simulink model "bike_model_v1_20190513_oldmodel"  (R2016b)
settings: Solver=ode23s  StartTime=0.0  StopTime=sim_time  FixedStep=Ts_IMU  MaxStep=Ts  RelTol=1e-3
values from neighbouring files (symbols this model uses):
  A = [0      0            1 ... (first row only)    [bike_init_v1_20190523_oldmodel_NOfeedback_RealModelComparison.m]    (also in bike_init_v1_20190524_oldmodel_positionfeedback_Nobalancing.m; bike_init_v1_20190527_oldmodel_NObalancing.m; bike_init_v1_20190527_oldmodel_positionfeedback_and_indicator.m; bike_init_v1_20190528_oldmodel_positionfeedback_and_indicator.m)
  B = [0; 1; (a_real*v*sin(lambda_real))/(h_real*b_real)]    [bike_init_v1_20190523_oldmodel_NOfeedback_RealModelComparison.m]    (also in bike_init_v1_20190524_oldmodel_positionfeedback_Nobalancing.m; bike_init_v1_20190527_oldmodel_NObalancing.m; bike_init_v1_20190527_oldmodel_positionfeedback_and_indicator.m; bike_init_v1_20190528_oldmodel_positionfeedback_and_indicator.m)
  b_model = 1.095*(1+(-0.1+(0.2*rand)))    [bike_init_v1_20190523_oldmodel_NOfeedback_RealModelComparison.m]    (also in bike_init_v1_20190524_oldmodel_positionfeedback_Nobalancing.m = 1.095; bike_init_v1_20190527_oldmodel_NObalancing.m = 1.095; bike_init_v1_20190527_oldmodel_positionfeedback_and_indicator.m = 1.095; bike_init_v1_20190528_oldmodel_positionfeedback_and_indicator.m = 1.095)
  b_real = 1.095    [bike_init_v1_20190523_oldmodel_NOfeedback_RealModelComparison.m]    (also in bike_init_v1_20190524_oldmodel_positionfeedback_Nobalancing.m; bike_init_v1_20190527_oldmodel_NObalancing.m; bike_init_v1_20190527_oldmodel_positionfeedback_and_indicator.m; bike_init_v1_20190528_oldmodel_positionfeedback_and_indicator.m)
  complementary = 0.985    [bike_init_v1_20190523_oldmodel_NOfeedback_RealModelComparison.m]    (also in bike_init_v1_20190524_oldmodel_positionfeedback_Nobalancing.m; bike_init_v1_20190527_oldmodel_NObalancing.m; bike_init_v1_20190527_oldmodel_positionfeedback_and_indicator.m; bike_init_v1_20190528_oldmodel_positionfeedback_and_indicator.m)
  cumulative_dist_along_path = [0;cumsum(dist_from_vertex_to_vertex,1)]    [bike_init_v1_20190523_oldmodel_NOfeedback_RealModelComparison.m]    (also in bike_init_v1_20190524_oldmodel_positionfeedback_Nobalancing.m; bike_init_v1_20190527_oldmodel_NObalancing.m; bike_init_v1_20190527_oldmodel_positionfeedback_and_indicator.m; bike_init_v1_20190528_oldmodel_positionfeedback_and_indicator.m)
  damp = 0.4    [bike_init_v1_20190523_oldmodel_NOfeedback_RealModelComparison.m]    (also in bike_init_v1_20190524_oldmodel_positionfeedback_Nobalancing.m; bike_init_v1_20190527_oldmodel_NObalancing.m; bike_init_v1_20190527_oldmodel_positionfeedback_and_indicator.m; bike_init_v1_20190528_oldmodel_positionfeedback_and_indicator.m)
  Dead_Band = [0.055,-0.055,0.005]    [bike_init_v1_20190523_oldmodel_NOfeedback_RealModelComparison.m]    (also in bike_init_v1_20190524_oldmodel_positionfeedback_Nobalancing.m; bike_init_v1_20190527_oldmodel_NObalancing.m; bike_init_v1_20190527_oldmodel_positionfeedback_and_indicator.m; bike_init_v1_20190528_oldmodel_positionfeedback_and_indicator.m)
  delay = 0.045    [bike_init_v1_20190523_oldmodel_NOfeedback_RealModelComparison.m]    (also in bike_init_v1_20190524_oldmodel_positionfeedback_Nobalancing.m; bike_init_v1_20190527_oldmodel_NObalancing.m; bike_init_v1_20190527_oldmodel_positionfeedback_and_indicator.m; bike_init_v1_20190528_oldmodel_positionfeedback_and_indicator.m)
  delta_control = 1    [bike_init_v1_20190523_oldmodel_NOfeedback_RealModelComparison.m]    (also in bike_init_v1_20190524_oldmodel_positionfeedback_Nobalancing.m; bike_init_v1_20190527_oldmodel_NObalancing.m; bike_init_v1_20190527_oldmodel_positionfeedback_and_indicator.m; bike_init_v1_20190528_oldmodel_positionfeedback_and_indicator.m)
  direct_control = 1    [bike_init_v1_20190523_oldmodel_NOfeedback_RealModelComparison.m]    (also in bike_init_v1_20190524_oldmodel_positionfeedback_Nobalancing.m; bike_init_v1_20190527_oldmodel_NObalancing.m; bike_init_v1_20190527_oldmodel_positionfeedback_and_indicator.m; bike_init_v1_20190528_oldmodel_positionfeedback_and_indicator.m)
  filter_model = 1    [bike_init_v1_20190523_oldmodel_NOfeedback_RealModelComparison.m]    (also in bike_init_v1_20190524_oldmodel_positionfeedback_Nobalancing.m; bike_init_v1_20190527_oldmodel_NObalancing.m; bike_init_v1_20190527_oldmodel_positionfeedback_and_indicator.m; bike_init_v1_20190528_oldmodel_positionfeedback_and_indicator.m)
  forward_motor_dynamics = 0    [bike_init_v1_20190523_oldmodel_NOfeedback_RealModelComparison.m]    (also in bike_init_v1_20190524_oldmodel_positionfeedback_Nobalancing.m; bike_init_v1_20190527_oldmodel_NObalancing.m; bike_init_v1_20190527_oldmodel_positionfeedback_and_indicator.m; bike_init_v1_20190528_oldmodel_positionfeedback_and_indicator.m)
  fr_oscil = 1    [bike_init_v1_20190523_oldmodel_NOfeedback_RealModelComparison.m]    (also in bike_init_v1_20190524_oldmodel_positionfeedback_Nobalancing.m; bike_init_v1_20190527_oldmodel_NObalancing.m; bike_init_v1_20190527_oldmodel_positionfeedback_and_indicator.m; bike_init_v1_20190528_oldmodel_positionfeedback_and_indicator.m)
  g = 9.81    [bike_init_v1_20190523_oldmodel_NOfeedback_RealModelComparison.m]    (also in bike_init_v1_20190524_oldmodel_positionfeedback_Nobalancing.m; bike_init_v1_20190527_oldmodel_NObalancing.m; bike_init_v1_20190527_oldmodel_positionfeedback_and_indicator.m; bike_init_v1_20190528_oldmodel_positionfeedback_and_indicator.m)
  gain = 0.3    [bike_init_v1_20190523_oldmodel_NOfeedback_RealModelComparison.m]    (also in bike_init_v1_20190524_oldmodel_positionfeedback_Nobalancing.m; bike_init_v1_20190527_oldmodel_NObalancing.m; bike_init_v1_20190527_oldmodel_positionfeedback_and_indicator.m; bike_init_v1_20190528_oldmodel_positionfeedback_and_indicator.m)
  IMU_height_model = 0.45*(1+(-0.1+(0.2*rand)))    [bike_init_v1_20190523_oldmodel_NOfeedback_RealModelComparison.m]    (also in bike_init_v1_20190524_oldmodel_positionfeedback_Nobalancing.m = 0.45; bike_init_v1_20190527_oldmodel_NObalancing.m = 0.45; bike_init_v1_20190527_oldmodel_positionfeedback_and_indicator.m = 0.45; bike_init_v1_20190528_oldmodel_positionfeedback_and_indicator.m = 0.45)
  IMU_height_real = 0.45    [bike_init_v1_20190523_oldmodel_NOfeedback_RealModelComparison.m]    (also in bike_init_v1_20190524_oldmodel_positionfeedback_Nobalancing.m; bike_init_v1_20190527_oldmodel_NObalancing.m; bike_init_v1_20190527_oldmodel_positionfeedback_and_indicator.m; bike_init_v1_20190528_oldmodel_positionfeedback_and_indicator.m)
  initial_states = [deg2rad(0) deg2rad(0) deg2rad(0)]    [bike_init_v1_20190523_oldmodel_NOfeedback_RealModelComparison.m]    (also in bike_init_v1_20190524_oldmodel_positionfeedback_Nobalancing.m; bike_init_v1_20190527_oldmodel_NObalancing.m; bike_init_v1_20190527_oldmodel_positionfeedback_and_indicator.m; bike_init_v1_20190528_oldmodel_positionfeedback_and_indicator.m = [deg2rad(1) deg2rad(0) deg2rad(0)])
  initial_x = path_x(1)+x_ini_diff    [bike_init_v1_20190523_oldmodel_NOfeedback_RealModelComparison.m]    (also in bike_init_v1_20190524_oldmodel_positionfeedback_Nobalancing.m; bike_init_v1_20190527_oldmodel_NObalancing.m; bike_init_v1_20190527_oldmodel_positionfeedback_and_indicator.m; bike_init_v1_20190528_oldmodel_positionfeedback_and_indicator.m)
  initial_y = radius+y_ini_diff    (= 20)    [bike_init_v1_20190523_oldmodel_NOfeedback_RealModelComparison.m]    (also in bike_init_v1_20190524_oldmodel_positionfeedback_Nobalancing.m; bike_init_v1_20190527_oldmodel_NObalancing.m; bike_init_v1_20190527_oldmodel_positionfeedback_and_indicator.m; bike_init_v1_20190528_oldmodel_positionfeedback_and_indicator.m)
  input_velocity = 2    [bike_init_v1_20190523_oldmodel_NOfeedback_RealModelComparison.m]    (also in bike_init_v1_20190524_oldmodel_positionfeedback_Nobalancing.m = 2.5; bike_init_v1_20190527_oldmodel_NObalancing.m = 2.5; bike_init_v1_20190527_oldmodel_positionfeedback_and_indicator.m = 3; bike_init_v1_20190528_oldmodel_positionfeedback_and_indicator.m = 7)
  K_full_dis = zeros(length(velocity_lqr),3)    [bike_init_v1_20190523_oldmodel_NOfeedback_RealModelComparison.m]    (also in bike_init_v1_20190524_oldmodel_positionfeedback_Nobalancing.m; bike_init_v1_20190527_oldmodel_NObalancing.m; bike_init_v1_20190527_oldmodel_positionfeedback_and_indicator.m; bike_init_v1_20190528_oldmodel_positionfeedback_and_indicator.m)
  lambda_model = deg2rad(70)*(1+(-0.1+(0.2*rand)))    [bike_init_v1_20190523_oldmodel_NOfeedback_RealModelComparison.m]    (also in bike_init_v1_20190524_oldmodel_positionfeedback_Nobalancing.m = deg2rad(70); bike_init_v1_20190527_oldmodel_NObalancing.m = deg2rad(70); bike_init_v1_20190527_oldmodel_positionfeedback_and_indicator.m = deg2rad(70); bike_init_v1_20190528_oldmodel_positionfeedback_and_indicator.m = deg2rad(70))
  lambda_real = deg2rad(70)    [bike_init_v1_20190523_oldmodel_NOfeedback_RealModelComparison.m]    (also in bike_init_v1_20190524_oldmodel_positionfeedback_Nobalancing.m; bike_init_v1_20190527_oldmodel_NObalancing.m; bike_init_v1_20190527_oldmodel_positionfeedback_and_indicator.m; bike_init_v1_20190528_oldmodel_positionfeedback_and_indicator.m)
  lat_control = 1    [bike_init_v1_20190523_oldmodel_NOfeedback_RealModelComparison.m]    (also in bike_init_v1_20190524_oldmodel_positionfeedback_Nobalancing.m; bike_init_v1_20190527_oldmodel_NObalancing.m; bike_init_v1_20190527_oldmodel_positionfeedback_and_indicator.m; bike_init_v1_20190528_oldmodel_positionfeedback_and_indicator.m)
  look_ahead = 0    [bike_init_v1_20190523_oldmodel_NOfeedback_RealModelComparison.m]    (also in bike_init_v1_20190524_oldmodel_positionfeedback_Nobalancing.m; bike_init_v1_20190527_oldmodel_NObalancing.m; bike_init_v1_20190527_oldmodel_positionfeedback_and_indicator.m; bike_init_v1_20190528_oldmodel_positionfeedback_and_indicator.m)
  max_handlebar = 40*(pi/180)    (= 0.698131700798)    [bike_init_v1_20190523_oldmodel_NOfeedback_RealModelComparison.m]    (also in bike_init_v1_20190524_oldmodel_positionfeedback_Nobalancing.m; bike_init_v1_20190527_oldmodel_NObalancing.m; bike_init_v1_20190527_oldmodel_positionfeedback_and_indicator.m; bike_init_v1_20190528_oldmodel_positionfeedback_and_indicator.m)
  max_roll = pi/2    (= 1.57079632679)    [bike_init_v1_20190523_oldmodel_NOfeedback_RealModelComparison.m]    (also in bike_init_v1_20190524_oldmodel_positionfeedback_Nobalancing.m; bike_init_v1_20190527_oldmodel_NObalancing.m; bike_init_v1_20190527_oldmodel_positionfeedback_and_indicator.m; bike_init_v1_20190528_oldmodel_positionfeedback_and_indicator.m)
  max_steering_motor_acc = inf    [bike_init_v1_20190523_oldmodel_NOfeedback_RealModelComparison.m]    (also in bike_init_v1_20190524_oldmodel_positionfeedback_Nobalancing.m; bike_init_v1_20190527_oldmodel_NObalancing.m; bike_init_v1_20190527_oldmodel_positionfeedback_and_indicator.m; bike_init_v1_20190528_oldmodel_positionfeedback_and_indicator.m)
  max_steering_motor_speed = 7.5    [bike_init_v1_20190523_oldmodel_NOfeedback_RealModelComparison.m]    (also in bike_init_v1_20190524_oldmodel_positionfeedback_Nobalancing.m; bike_init_v1_20190527_oldmodel_NObalancing.m; bike_init_v1_20190527_oldmodel_positionfeedback_and_indicator.m; bike_init_v1_20190528_oldmodel_positionfeedback_and_indicator.m)
  min_handlebar = -max_handlebar    (= -0.698131700798)    [bike_init_v1_20190523_oldmodel_NOfeedback_RealModelComparison.m]    (also in bike_init_v1_20190524_oldmodel_positionfeedback_Nobalancing.m; bike_init_v1_20190527_oldmodel_NObalancing.m; bike_init_v1_20190527_oldmodel_positionfeedback_and_indicator.m; bike_init_v1_20190528_oldmodel_positionfeedback_and_indicator.m)
  min_roll = - max_roll    (= -1.57079632679)    [bike_init_v1_20190523_oldmodel_NOfeedback_RealModelComparison.m]    (also in bike_init_v1_20190524_oldmodel_positionfeedback_Nobalancing.m; bike_init_v1_20190527_oldmodel_NObalancing.m; bike_init_v1_20190527_oldmodel_positionfeedback_and_indicator.m; bike_init_v1_20190528_oldmodel_positionfeedback_and_indicator.m)
  min_steering_motor_acc = -inf    [bike_init_v1_20190523_oldmodel_NOfeedback_RealModelComparison.m]    (also in bike_init_v1_20190524_oldmodel_positionfeedback_Nobalancing.m; bike_init_v1_20190527_oldmodel_NObalancing.m; bike_init_v1_20190527_oldmodel_positionfeedback_and_indicator.m; bike_init_v1_20190528_oldmodel_positionfeedback_and_indicator.m)
  min_steering_motor_speed = -7.5    [bike_init_v1_20190523_oldmodel_NOfeedback_RealModelComparison.m]    (also in bike_init_v1_20190524_oldmodel_positionfeedback_Nobalancing.m; bike_init_v1_20190527_oldmodel_NObalancing.m; bike_init_v1_20190527_oldmodel_positionfeedback_and_indicator.m; bike_init_v1_20190528_oldmodel_positionfeedback_and_indicator.m)
  noise = 1    [bike_init_v1_20190523_oldmodel_NOfeedback_RealModelComparison.m]    (also in bike_init_v1_20190524_oldmodel_positionfeedback_Nobalancing.m; bike_init_v1_20190527_oldmodel_NObalancing.m; bike_init_v1_20190527_oldmodel_positionfeedback_and_indicator.m; bike_init_v1_20190528_oldmodel_positionfeedback_and_indicator.m)
  noise_encoder = 1e-7    (= 1e-07)    [bike_init_v1_20190523_oldmodel_NOfeedback_RealModelComparison.m]    (also in bike_init_v1_20190524_oldmodel_positionfeedback_Nobalancing.m; bike_init_v1_20190527_oldmodel_NObalancing.m; bike_init_v1_20190527_oldmodel_positionfeedback_and_indicator.m; bike_init_v1_20190528_oldmodel_positionfeedback_and_indicator.m)
  noise_hall = 0    [bike_init_v1_20190523_oldmodel_NOfeedback_RealModelComparison.m]    (also in bike_init_v1_20190524_oldmodel_positionfeedback_Nobalancing.m = 0.01; bike_init_v1_20190527_oldmodel_NObalancing.m; bike_init_v1_20190527_oldmodel_positionfeedback_and_indicator.m = 0.01; bike_init_v1_20190528_oldmodel_positionfeedback_and_indicator.m = 0.01)
  oscillations_roll = 0    [bike_init_v1_20190523_oldmodel_NOfeedback_RealModelComparison.m]    (also in bike_init_v1_20190524_oldmodel_positionfeedback_Nobalancing.m; bike_init_v1_20190527_oldmodel_NObalancing.m; bike_init_v1_20190527_oldmodel_positionfeedback_and_indicator.m; bike_init_v1_20190528_oldmodel_positionfeedback_and_indicator.m)
  oscillations_steer = 0    [bike_init_v1_20190523_oldmodel_NOfeedback_RealModelComparison.m]    (also in bike_init_v1_20190524_oldmodel_positionfeedback_Nobalancing.m; bike_init_v1_20190527_oldmodel_NObalancing.m; bike_init_v1_20190527_oldmodel_positionfeedback_and_indicator.m; bike_init_v1_20190528_oldmodel_positionfeedback_and_indicator.m)
  parameters_model = [g h_model b_model a_model lambda_model c_model]    [bike_init_v1_20190523_oldmodel_NOfeedback_RealModelComparison.m]    (also in bike_init_v1_20190524_oldmodel_positionfeedback_Nobalancing.m; bike_init_v1_20190527_oldmodel_NObalancing.m; bike_init_v1_20190527_oldmodel_positionfeedback_and_indicator.m; bike_init_v1_20190528_oldmodel_positionfeedback_and_indicator.m)
  parameters_real = [g h_real b_real a_real lambda_real c_real]    [bike_init_v1_20190523_oldmodel_NOfeedback_RealModelComparison.m]    (also in bike_init_v1_20190524_oldmodel_positionfeedback_Nobalancing.m; bike_init_v1_20190527_oldmodel_NObalancing.m; bike_init_v1_20190527_oldmodel_positionfeedback_and_indicator.m; bike_init_v1_20190528_oldmodel_positionfeedback_and_indicator.m)
  path_tracking = 1    [bike_init_v1_20190523_oldmodel_NOfeedback_RealModelComparison.m]    (also in bike_init_v1_20190524_oldmodel_positionfeedback_Nobalancing.m; bike_init_v1_20190527_oldmodel_NObalancing.m; bike_init_v1_20190527_oldmodel_positionfeedback_and_indicator.m; bike_init_v1_20190528_oldmodel_positionfeedback_and_indicator.m = 0)
  path_x = [path_x1 path_x2 path_x3]    [bike_init_v1_20190523_oldmodel_NOfeedback_RealModelComparison.m]    (also in bike_init_v1_20190524_oldmodel_positionfeedback_Nobalancing.m; bike_init_v1_20190527_oldmodel_NObalancing.m; bike_init_v1_20190527_oldmodel_positionfeedback_and_indicator.m; bike_init_v1_20190528_oldmodel_positionfeedback_and_indicator.m)
  path_y = [path_y1 path_y2 path_y3]    [bike_init_v1_20190523_oldmodel_NOfeedback_RealModelComparison.m]    (also in bike_init_v1_20190524_oldmodel_positionfeedback_Nobalancing.m; bike_init_v1_20190527_oldmodel_NObalancing.m; bike_init_v1_20190527_oldmodel_positionfeedback_and_indicator.m; bike_init_v1_20190528_oldmodel_positionfeedback_and_indicator.m)
  plant_model = 1    [bike_init_v1_20190523_oldmodel_NOfeedback_RealModelComparison.m]    (also in bike_init_v1_20190524_oldmodel_positionfeedback_Nobalancing.m; bike_init_v1_20190527_oldmodel_NObalancing.m; bike_init_v1_20190527_oldmodel_positionfeedback_and_indicator.m; bike_init_v1_20190528_oldmodel_positionfeedback_and_indicator.m)
  roll_rate_coef = 0.9    [bike_init_v1_20190523_oldmodel_NOfeedback_RealModelComparison.m]    (also in bike_init_v1_20190524_oldmodel_positionfeedback_Nobalancing.m; bike_init_v1_20190527_oldmodel_NObalancing.m; bike_init_v1_20190527_oldmodel_positionfeedback_and_indicator.m; bike_init_v1_20190528_oldmodel_positionfeedback_and_indicator.m)
  sensordist = dout*pi/nrsensor    (= 0.439822971503)    [bike_init_v1_20190524_oldmodel_positionfeedback_Nobalancing.m]    (also in bike_init_v1_20190527_oldmodel_NObalancing.m; bike_init_v1_20190527_oldmodel_positionfeedback_and_indicator.m; bike_init_v1_20190528_oldmodel_positionfeedback_and_indicator.m; bike_init_v1_20190531_oldmodel_positionfeedback_and_indicator.m)
  steering_motor_limitations = 1    [bike_init_v1_20190523_oldmodel_NOfeedback_RealModelComparison.m]    (also in bike_init_v1_20190524_oldmodel_positionfeedback_Nobalancing.m; bike_init_v1_20190527_oldmodel_NObalancing.m; bike_init_v1_20190527_oldmodel_positionfeedback_and_indicator.m; bike_init_v1_20190528_oldmodel_positionfeedback_and_indicator.m)
  sys_con = ss(A,B,C,D)    [bike_init_v1_20190523_oldmodel_NOfeedback_RealModelComparison.m]    (also in bike_init_v1_20190524_oldmodel_positionfeedback_Nobalancing.m; bike_init_v1_20190527_oldmodel_NObalancing.m; bike_init_v1_20190527_oldmodel_positionfeedback_and_indicator.m; bike_init_v1_20190528_oldmodel_positionfeedback_and_indicator.m)
  sys_dis = c2d(sys_con,Ts)    [bike_init_v1_20190523_oldmodel_NOfeedback_RealModelComparison.m]    (also in bike_init_v1_20190524_oldmodel_positionfeedback_Nobalancing.m; bike_init_v1_20190527_oldmodel_NObalancing.m; bike_init_v1_20190527_oldmodel_positionfeedback_and_indicator.m; bike_init_v1_20190528_oldmodel_positionfeedback_and_indicator.m)
  ToleranceVelocityEst = 0.5    [bike_init_v1_20190524_oldmodel_positionfeedback_Nobalancing.m]    (also in bike_init_v1_20190527_oldmodel_NObalancing.m; bike_init_v1_20190527_oldmodel_positionfeedback_and_indicator.m; bike_init_v1_20190528_oldmodel_positionfeedback_and_indicator.m; bike_init_v1_20190531_oldmodel_positionfeedback_and_indicator.m)
  Ts = 0.04    [bike_init_v1_20190523_oldmodel_NOfeedback_RealModelComparison.m]    (also in bike_init_v1_20190524_oldmodel_positionfeedback_Nobalancing.m; bike_init_v1_20190527_oldmodel_NObalancing.m; bike_init_v1_20190527_oldmodel_positionfeedback_and_indicator.m; bike_init_v1_20190528_oldmodel_positionfeedback_and_indicator.m)
  Ts_IMU = 0.04    [bike_init_v1_20190523_oldmodel_NOfeedback_RealModelComparison.m]    (also in bike_init_v1_20190524_oldmodel_positionfeedback_Nobalancing.m; bike_init_v1_20190527_oldmodel_NObalancing.m; bike_init_v1_20190527_oldmodel_positionfeedback_and_indicator.m; bike_init_v1_20190528_oldmodel_positionfeedback_and_indicator.m)
  velocity_lqr = [velocity_lqr-0.1 velocity_lqr velocity_lqr+0.1]    [bike_init_v1_20190523_oldmodel_NOfeedback_RealModelComparison.m]    (also in bike_init_v1_20190524_oldmodel_positionfeedback_Nobalancing.m; bike_init_v1_20190527_oldmodel_NObalancing.m; bike_init_v1_20190527_oldmodel_positionfeedback_and_indicator.m; bike_init_v1_20190528_oldmodel_positionfeedback_and_indicator.m)
  velocity_wave_amp = 0.5    [bike_init_v1_20190523_oldmodel_NOfeedback_RealModelComparison.m]    (also in bike_init_v1_20190524_oldmodel_positionfeedback_Nobalancing.m; bike_init_v1_20190527_oldmodel_NObalancing.m; bike_init_v1_20190527_oldmodel_positionfeedback_and_indicator.m; bike_init_v1_20190528_oldmodel_positionfeedback_and_indicator.m)
  velocity_wave_freq = 0.3*2*pi    (= 1.88495559215)    [bike_init_v1_20190523_oldmodel_NOfeedback_RealModelComparison.m]    (also in bike_init_v1_20190524_oldmodel_positionfeedback_Nobalancing.m; bike_init_v1_20190527_oldmodel_NObalancing.m; bike_init_v1_20190527_oldmodel_positionfeedback_and_indicator.m; bike_init_v1_20190528_oldmodel_positionfeedback_and_indicator.m)
undefined symbols (not defined in the file or in its folder): curvature
libraries: simulink x13, dspsigops x2, simulink_extras x1
(part 1 of 3)
settings Model: Creator=Boaz Ash  LastModifiedBy=maximefeingesicht
settings DebuggingCC: UnconnectedInputMsg=none  UnconnectedOutputMsg=none  UnconnectedLineMsg=none

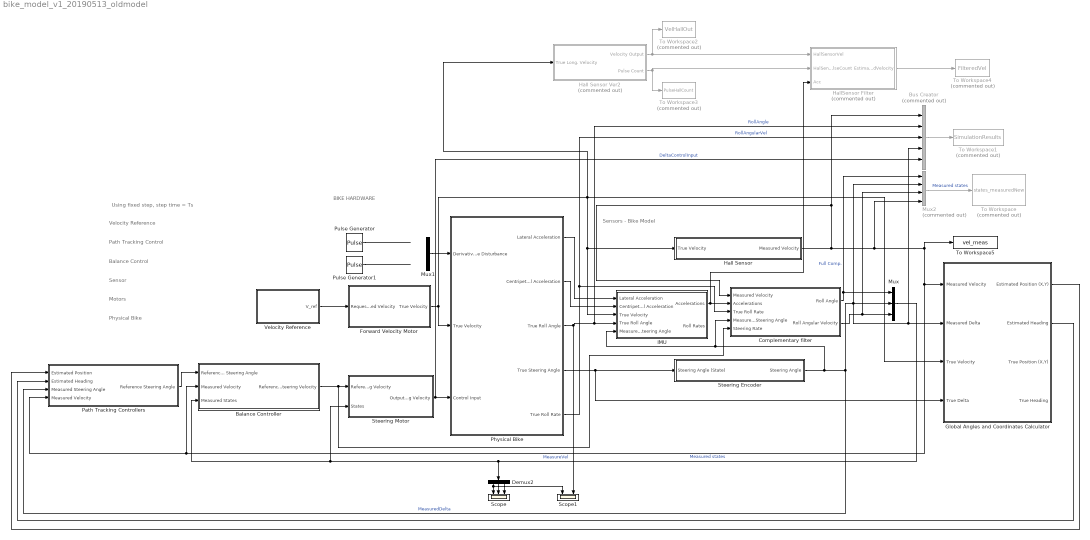
== system bike_model_v1_20190513_oldmodel ==
  note: Using fixed step, step time = Ts
  note: BIKE HARDWARE
  note: Velocity Reference
  note: Sensor
  note: Sensors - Bike Model
  note: Balance Control
  note: Motors
  note: Physical Bike
  note: Path Tracking Control
  Balance Controller : Subsystem  TreatAsAtomicUnit=on  SystemSampleTime=Ts
  Bus Creator : BusCreator  Commented=on  Inputs=5
  Complementary filter : Subsystem  SystemSampleTime=Ts_IMU
  Demux2 : Demux  Outputs=3
  Forward Velocity Motor : Subsystem
  Global Angles and Coordinates Calculator : Subsystem  SystemSampleTime=Ts
  Hall Sensor : Subsystem  TreatAsAtomicUnit=on  SystemSampleTime=Ts
  Hall Sensor Ver2 : Subsystem  Commented=on
  HallSensor Filter : Subsystem  Commented=on
  IMU : Subsystem  TreatAsAtomicUnit=on
  Mux : Mux  Inputs=3
  Mux1 : Mux  Inputs=3
  Mux2 : Mux  Commented=on
  Path Tracking Controllers : Subsystem
  Physical Bike : Subsystem
  Pulse Generator : DiscretePulseGenerator  PulseType=Time based  Amplitude=pi/36  Period=100  PhaseDelay=1
  Pulse Generator1 : DiscretePulseGenerator  PulseType=Time based  Amplitude=-deg2rad(30)  Period=10  PulseWidth=10  PhaseDelay=1
  Scope : Scope  NumInputPorts=3
  Scope1 : Scope  NumInputPorts=2
  Steering Encoder : Subsystem  TreatAsAtomicUnit=on  SystemSampleTime=Ts
  Steering Motor : Subsystem
  To Workspace : ToWorkspace  Commented=on  VariableName=states_measuredNew  SaveFormat=Timeseries  SampleTime=-1
  To Workspace1 : ToWorkspace  Commented=on  VariableName=SimulationResults  SaveFormat=Timeseries  SampleTime=-1
      settings: Decimation=2  Save2DSignal=2-D array (concatenate along first dimension)
  To Workspace2 : ToWorkspace  Commented=on  VariableName=VelHallOut  SaveFormat=Timeseries  SampleTime=Ts
  To Workspace3 : ToWorkspace  Commented=on  VariableName=PulseHallCount  SaveFormat=Timeseries  SampleTime=Ts
  To Workspace4 : ToWorkspace  Commented=on  VariableName=FilteredVel  SaveFormat=Timeseries  SampleTime=-1
  To Workspace5 : ToWorkspace  VariableName=vel_meas  SaveFormat=Timeseries  SampleTime=-1
  Velocity Reference : Subsystem
  wires:
  Complementary filter/1(Roll Angle) -> Mux2/1, Mux/1  "Full Comp."
  Complementary filter/2(Roll Angular Velocity) -> Mux2/3, Mux/3
  Mux1/1 -> Physical Bike/1(Derivative Disturbance)
  Velocity Reference/1(V_ref) -> Forward Velocity Motor/1(Requested Velocity)
  Demux2/2 -> Scope/2
  Demux2/3 -> Scope/3
  Forward Velocity Motor/1(True Velocity) -> Hall Sensor/1(True Velocity), IMU/3(True Velocity), Hall Sensor Ver2/1(True Long. Velocity), Global Angles and Coordinates Calculator/3(True Velocity), Physical Bike/2(True Velocity)
  Pulse Generator/1 -> ?
  Physical Bike/4(True Steering Angle) -> Global Angles and Coordinates Calculator/4(True Delta), Steering Encoder/1(Steering Angle (State))
  Pulse Generator1/1 -> ?
  Global Angles and Coordinates Calculator/1(Estimated Position (X,Y)) -> Path Tracking Controllers/1(Estimated Position)
  Global Angles and Coordinates Calculator/2(Estimated Heading) -> Path Tracking Controllers/2(Estimated Heading)
  Path Tracking Controllers/1(Reference Steering Angle) -> Balance Controller/1(Reference Steering Angle)
  Balance Controller/1(Reference Steering Velocity) -> Complementary filter/5(Steering Rate), Steering Motor/1(Reference Steering Velocity)
  Demux2/1 -> Scope1/1, Scope/1
  Physical Bike/1(Lateral Acceleration) -> IMU/1(Lateral Acceleration)
  Physical Bike/2(Centripetal Acceleration) -> IMU/2(Centripetal Acceleration)
  Mux2/1 -> To Workspace/1  "Measured states"
  Mux/1 -> Demux2/1, Steering Motor/2(States), Balance Controller/3(Measured States)  "Measured states"
  HallSensor Filter/1(EstimatedVelocity) -> To Workspace4/1
  Bus Creator/1 -> To Workspace1/1
  Hall Sensor/1(Measured Velocity) -> Bus Creator/1, Complementary filter/1(Measured Velocity), To Workspace5/1, Path Tracking Controllers/4(Measured Velocity), Balance Controller/2(Measured Velocity), Global Angles and Coordinates Calculator/1(Measured Velocity), Mux2/4  "MeasureVel"
  Physical Bike/5(True Roll Rate) -> Bus Creator/3, Complementary filter/3(True Roll Rate)  "RollAngularVel"
  Hall Sensor Ver2/1(Velocity Output) -> To Workspace2/1, HallSensor Filter/1(HallSensorVel)
  Physical Bike/3(True Roll Angle) -> Bus Creator/2, IMU/4(True Roll Angle), Scope1/2  "RollAngle"
  Steering Motor/1(Output Steering Velocity) -> Bus Creator/5, Physical Bike/3(Control Input)  "DeltaControlInput"
  Hall Sensor Ver2/2(" Pulse Count") -> HallSensor Filter/2(HalSensorPulseCount), To Workspace3/1
  Steering Encoder/1(Steering Angle) -> IMU/5(Measured Steering Angle), Complementary filter/4(Measured Steering Angle), Global Angles and Coordinates Calculator/2(Measured Delta), Bus Creator/4, Mux2/2, Mux/2, Path Tracking Controllers/3(Measured Steering Angle)  "MeasuredDelta"
  IMU/1(Accelerations) -> HallSensor Filter/3(Acc), Complementary filter/2(Accelerations)

== system bike_model_v1_20190513_oldmodel/Balance Controller ==
  Reference Steering Angle : Inport
  Measured Velocity : Inport  Port=2
  Measured States : Inport  Port=3
  LQR Controller : Subsystem  TreatAsAtomicUnit=on  SystemSampleTime=Ts
  Reference States : Subsystem  SystemSampleTime=Ts
  Sum : Sum  Inputs=|+-
  To Workspace : ToWorkspace  VariableName=states_measured  SaveFormat=Timeseries  SampleTime=-1
  Reference Steering Velocity : Outport
  wires:
  Reference States/1(Reference States) -> Sum/1
  Sum/1 -> LQR Controller/2(State Error)
  LQR Controller/1(Calculated Input) -> Reference Steering Velocity/1
  Reference Steering Angle/1 -> Reference States/2(Delta Ref)
  Measured Velocity/1 -> Reference States/1(Velocity), LQR Controller/1(Velocity)
  Measured States/1 -> To Workspace/1, Sum/2

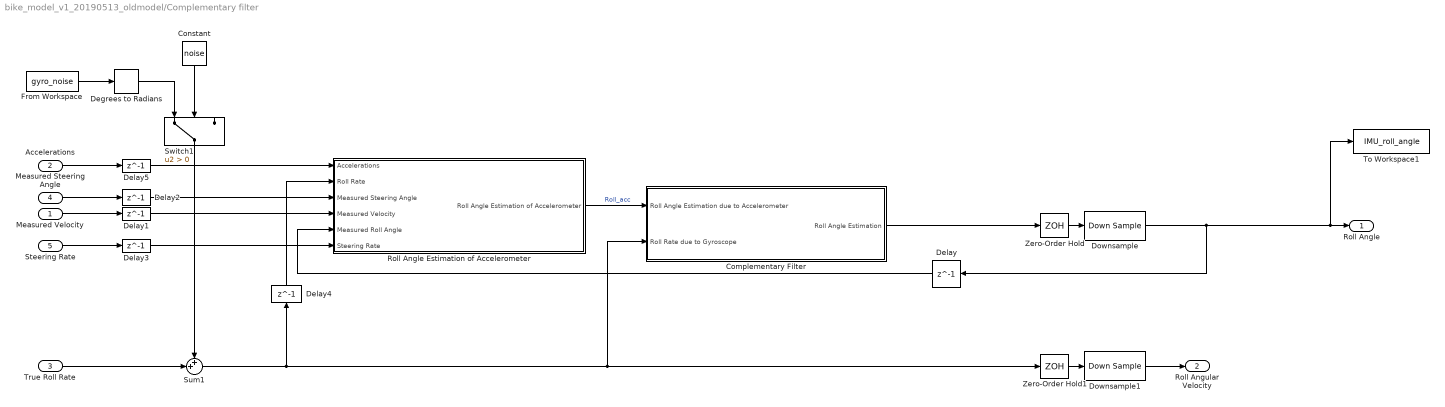
== system bike_model_v1_20190513_oldmodel/Complementary filter ==
  Measured Velocity : Inport
  Accelerations : Inport  Port=2
  True Roll Rate : Inport  Port=3
  Measured Steering Angle : Inport  Port=4
  Steering Rate : Inport  Port=5
  Complementary Filter : Subsystem  TreatAsAtomicUnit=on  SystemSampleTime=Ts_IMU
  Constant : Constant  Value=noise
  Degrees to Radians : simulink_extras/Transformations/Degrees to Radians
  Delay{,1..2,4..5} (5 alike) : Delay  DelayLength=1
  Delay3 : Delay  DelayLength=1  SampleTime=Ts_IMU
  Downsample : DownSample  N=Ts/Ts_IMU  RateOptions=Allow multirate processing
  Downsample1 : DownSample  N=Ts/Ts_IMU  RateOptions=Allow multirate processing
  From Workspace : FromWorkspace  VariableName=gyro_noise  SampleTime=0
  Roll Angle Estimation of Accelerometer : Subsystem
  Sum1 : Sum  Inputs=++|
  Switch1 : Switch  Criteria=u2 > Threshold
  To Workspace1 : ToWorkspace  VariableName=IMU_roll_angle  SaveFormat=Structure  SampleTime=-1
  Zero-Order Hold : ZeroOrderHold  SampleTime=Ts_IMU
  Zero-Order Hold1 : ZeroOrderHold  SampleTime=Ts_IMU
  Roll Angle : Outport
  Roll Angular Velocity : Outport  Port=2
  wires:
  Constant/1 -> Switch1/2
  True Roll Rate/1 -> Sum1/2
  Roll Angle Estimation of Accelerometer/1(Roll Angle Estimation of Accelerometer) -> Complementary Filter/1(Roll Angle Estimation due to Accelerometer)  "Roll_acc"
  Switch1/1 -> Sum1/1
  Sum1/1 -> Zero-Order Hold1/1, Complementary Filter/2(Roll Rate due to Gyroscope), Delay4/1
  Zero-Order Hold/1 -> Downsample/1
  Zero-Order Hold1/1 -> Downsample1/1
  Accelerations/1 -> Delay5/1
  Measured Steering Angle/1 -> Delay2/1
  Measured Velocity/1 -> Delay1/1
  Delay/1 -> Roll Angle Estimation of Accelerometer/5(Measured Roll Angle)
  Delay1/1 -> Roll Angle Estimation of Accelerometer/4(Measured Velocity)
  Delay2/1 -> Roll Angle Estimation of Accelerometer/3(Measured Steering Angle)
  Steering Rate/1 -> Delay3/1
  Delay3/1 -> Roll Angle Estimation of Accelerometer/6(Steering Rate)
  Delay4/1 -> Roll Angle Estimation of Accelerometer/2(Roll Rate)
  Delay5/1 -> Roll Angle Estimation of Accelerometer/1(Accelerations)
  Complementary Filter/1(Roll Angle Estimation) -> Zero-Order Hold/1
  From Workspace/1 -> Degrees to Radians/1
  Degrees to Radians/1 -> Switch1/1
  Downsample1/1 -> Roll Angular Velocity/1
  Downsample/1 -> To Workspace1/1, Roll Angle/1, Delay/1

== system bike_model_v1_20190513_oldmodel/Forward Velocity Motor ==
  note: Add limit for acceleration/deceleration
      | Add min speed of 1.69 m/s (3600 rpm motor speed) limitation
      | Add min speed of 8.20 m/s (18000 rpm motor speed) limitation
      | Add deadband and delay
  Requested Velocity : Inport
  Constant : Constant  Value=forward_motor_dynamics
  Rate Limiter : RateLimiter  RisingSlewLimit=inf  FallingSlewLimit=-inf  SampleTimeMode=inherited
  Saturation : Saturate  UpperLimit=inf  LowerLimit=0
  Scope : Scope
  Sine Wave : Sin  Amplitude=velocity_wave_amp  Frequency=velocity_wave_freq  SampleTime=0
  Sum : Sum  Inputs=|++
  Switch : Switch  Criteria=u2 > Threshold
  Transfer Fcn : TransferFcn  Numerator=[-0.2156 0.556]  Denominator=[1 1.675 0.5558]
  True Velocity : Outport
  wires:
  Requested Velocity/1 -> Transfer Fcn/1, Switch/3
  Transfer Fcn/1 -> Rate Limiter/1
  Switch/1 -> Sum/1
  Constant/1 -> Switch/2
  Saturation/1 -> Switch/1
  Rate Limiter/1 -> Saturation/1
  Sum/1 -> Scope/1, True Velocity/1
  Sine Wave/1 -> Sum/2

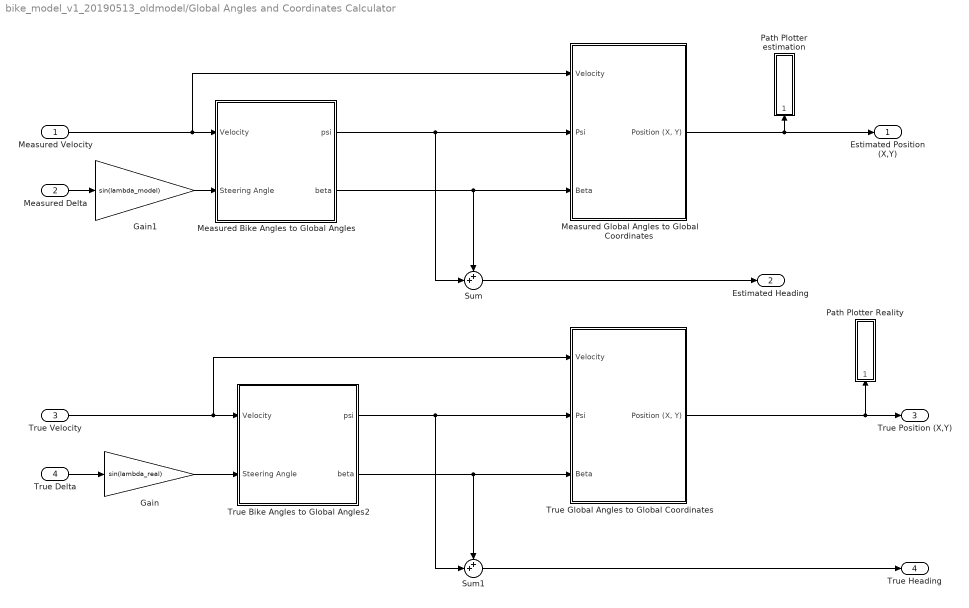
== system bike_model_v1_20190513_oldmodel/Global Angles and Coordinates Calculator ==
  Measured Velocity : Inport
  Measured Delta : Inport  Port=2
  True Velocity : Inport  Port=3
  True Delta : Inport  Port=4
  Gain : Gain  Gain=sin(lambda_real)
  Gain1 : Gain  Gain=sin(lambda_model)
  Measured Bike Angles to Global Angles : Subsystem
  Measured Global Angles to Global Coordinates : Subsystem
  Path Plotter Reality : Subsystem  SystemSampleTime=Ts
  Path Plotter estimation : Subsystem  SystemSampleTime=Ts
  Sum : Sum  Inputs=++|
  Sum1 : Sum  Inputs=++|
  True Bike Angles to Global Angles2 : Subsystem
  True Global Angles to Global Coordinates : Subsystem
  Estimated Position (X,Y) : Outport
  Estimated Heading : Outport  Port=2
  True Position (X,Y) : Outport  Port=3
  True Heading : Outport  Port=4
  wires:
  Measured Velocity/1 -> Measured Bike Angles to Global Angles/1(Velocity), Measured Global Angles to Global Coordinates/1(Velocity)
  Measured Bike Angles to Global Angles/1(psi) -> Sum/2, Measured Global Angles to Global Coordinates/2(Psi)
  True Global Angles to Global Coordinates/1("Position (X, Y)") -> Path Plotter Reality/1(Position), True Position (X,Y)/1
  True Delta/1 -> Gain/1
  True Velocity/1 -> True Global Angles to Global Coordinates/1(Velocity), True Bike Angles to Global Angles2/1(Velocity)
  Measured Bike Angles to Global Angles/2(beta) -> Measured Global Angles to Global Coordinates/3(Beta), Sum/1
  Measured Delta/1 -> Gain1/1
  Sum/1 -> Estimated Heading/1
  Sum1/1 -> True Heading/1
  True Bike Angles to Global Angles2/1(psi) -> Sum1/2, True Global Angles to Global Coordinates/2(Psi)
  True Bike Angles to Global Angles2/2(beta) -> Sum1/1, True Global Angles to Global Coordinates/3(Beta)
  Gain/1 -> True Bike Angles to Global Angles2/2(Steering Angle)
  Gain1/1 -> Measured Bike Angles to Global Angles/2(Steering Angle)
  Measured Global Angles to Global Coordinates/1("Position (X, Y)") -> Path Plotter estimation/1(Position), Estimated Position (X,Y)/1

== system bike_model_v1_20190513_oldmodel/Hall Sensor ==
  True Velocity : Inport
  Constant : Constant  Value=noise
  Noise on hall sensor : RandomNumber  Variance=noise_hall  Seed=1  SampleTime=Ts
  Saturate Signal : Switch  Criteria=u2 > Threshold
  Sum : Sum  Inputs=++|
  Switch : Switch  Criteria=u2 > Threshold
  Velocity Lower Bound : simulink/Model Verification/Check Static  Lower Bound  Description=0.6 <= u  min=0.6  min_included=on  enabled=on  stopWhenAssertionFail=off  export=on  icon=graphic
  Zero : Constant  Value=0
  Zero-Order Hold : ZeroOrderHold  SampleTime=Ts
  Measured Velocity : Outport
  wires:
  True Velocity/1 -> Sum/2, Switch/3
  Constant/1 -> Switch/2
  Switch/1 -> Saturate Signal/1, Velocity Lower Bound/1
  Noise on hall sensor/1 -> Sum/1
  Sum/1 -> Switch/1
  Zero/1 -> Saturate Signal/3
  Velocity Lower Bound/1 -> Saturate Signal/2
  Saturate Signal/1 -> Zero-Order Hold/1
  Zero-Order Hold/1 -> Measured Velocity/1

== system bike_model_v1_20190513_oldmodel/Hall Sensor Ver2 ==
  True Long. Velocity : Inport
  Clock : Clock
      settings: Decimation=3
  Delay : Delay  DelayLength=1  InitialCondition=0
  Distance Calculator : Integrator
  MATLAB Function : MATLAB Function  TreatAsAtomicUnit=on  SystemSampleTime=0.01
  MATLAB Function1 : MATLAB Function  Commented=on  TreatAsAtomicUnit=on
  MATLAB Function2 : MATLAB Function  Commented=on  TreatAsAtomicUnit=on  SystemSampleTime=0.01
      settings: MinAlgLoopOccurrences=on
  To Workspace : ToWorkspace  VariableName=PulseCount  SaveFormat=Timeseries  SampleTime=Ts
  To Workspace1 : ToWorkspace  VariableName=TrueDistance  SaveFormat=Timeseries  SampleTime=Ts
  sensor distances : Constant  Value=sensordist
  sensor distances1 : Constant  Commented=on  Value=sensordist
  Velocity Output : Outport
  " Pulse Count" : Outport  Port=2
  wires:
  MATLAB Function/1(Vout) -> Velocity Output/1
  Delay/1 -> MATLAB Function/3(count)
  Distance Calculator/1 -> To Workspace1/1, MATLAB Function/1(Dist)
  True Long. Velocity/1 -> Distance Calculator/1
  sensor distances/1 -> MATLAB Function/2(hallsensor_dist)
  Clock/1 -> MATLAB Function/4(T)
  MATLAB Function/3(newcount_output) -> To Workspace/1, Delay/1, " Pulse Count"/1
  sensor distances1/1 -> MATLAB Function1/2(SensorDist)

== system bike_model_v1_20190513_oldmodel/HallSensor Filter ==
  HallSensorVel : Inport
  HalSensorPulseCount : Inport  Port=2
  Acc : Inport  Port=3
  Complementary Filter Hall Sensor : MATLAB Function  TreatAsAtomicUnit=on  SystemSampleTime=Ts_IMU
  Constant : Constant  Value=Ts_IMU
  Constant1 : Constant  Value=ToleranceVelocityEst
  Demux : Demux  Outputs=3
  EstimatedVelocity : Outport
  wires:
  Complementary Filter Hall Sensor/1(EstimatedVelocity) -> EstimatedVelocity/1
  Constant/1 -> Complementary Filter Hall Sensor/4(T)
  HalSensorPulseCount/1 -> Complementary Filter Hall Sensor/2(PulseCount)
  Acc/1 -> Demux/1
  HallSensorVel/1 -> Complementary Filter Hall Sensor/1(HalVel)
  Demux/1 -> Complementary Filter Hall Sensor/3(Accx)
  Constant1/1 -> Complementary Filter Hall Sensor/5(Toler)

== system bike_model_v1_20190513_oldmodel/IMU ==
  Lateral Acceleration : Inport
  Centripetal Acceleration : Inport  Port=2
  True Velocity : Inport  Port=3
  True Roll Angle : Inport  Port=4
  Measured Steering Angle : Inport  Port=5
  IMU : Subsystem
  Accelerations : Outport
  Roll Rates : Outport  Port=2
  wires:
  True Velocity/1 -> IMU/3(True Velocity)
  True Roll Angle/1 -> IMU/4(True Roll Angle)
  Measured Steering Angle/1 -> IMU/5(Measured Steering Angle)
  Lateral Acceleration/1 -> IMU/1(Lateral Acceleration)
  Centripetal Acceleration/1 -> IMU/2(Centripetal Acceleration)
  IMU/1(Accelerations) -> Accelerations/1
  IMU/2(Roll Rates) -> Roll Rates/1

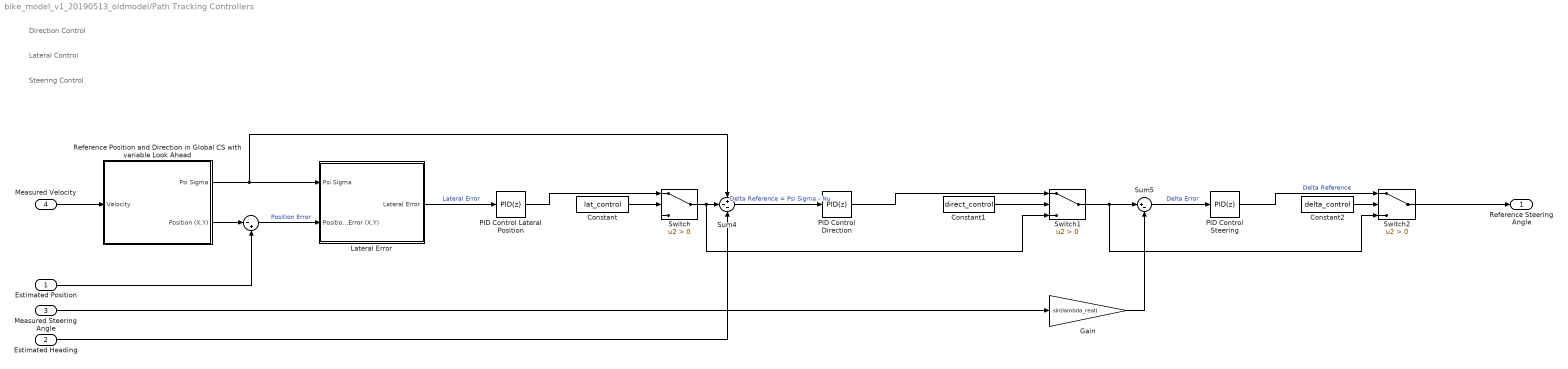
== system bike_model_v1_20190513_oldmodel/Path Tracking Controllers ==
  note: Direction Control
  note: Lateral Control
  note: Steering Control
  Estimated Position : Inport
  Estimated Heading : Inport  Port=2
  Measured Steering Angle : Inport  Port=3
  Measured Velocity : Inport  Port=4
  " " : Sum  Inputs=|-+
  Constant : Constant  Value=lat_control
  Constant1 : Constant  Value=direct_control
  Constant2 : Constant  Value=delta_control
  Gain : Gain  Gain=sin(lambda_real)
  Lateral Error : Subsystem  SystemSampleTime=Ts
  PID Control Lateral Position : simulink/Continuous/PID Controller  Controller=PID  TimeDomain=Discrete-time  SampleTime=Ts  IntegratorMethod=Forward Euler  FilterMethod=Forward Euler  Form=Parallel  UseFilter=on  ControllerParametersSource=internal  P=0.2  I=0.01  D=0  N=100  InitialConditionSource=internal  InitialConditionForIntegrator=0  InitialConditionForFilter=0  ExternalReset=none  LimitOutput=off  UpperSaturationLimit=inf  LowerSaturationLimit=-inf  LinearizeAsGain=on  AntiWindupMode=none  Kb=1  TrackingMode=off  Kt=1  PParamMin=[]  PParamMax=[]  IParamMin=[]  IParamMax=[]  DParamMin=[]  DParamMax=[]  NParamMin=[]  NParamMax=[]  KbParamMin=[]  KbParamMax=[]  KtParamMin=[]  KtParamMax=[]  POutMin=[]  POutMax=[]  IOutMin=[]  IOutMax=[]  DOutMin=[]  DOutMax=[]  NOutMin=[]  NOutMax=[]  KbOutMin=[]  KbOutMax=[]  KtOutMin=[]  KtOutMax=[]  IntegratorOutMin=[]  IntegratorOutMax=[]  FilterOutMin=[]  FilterOutMax=[]  SumOutMin=[]  SumOutMax=[]  SumI1OutMin=[]  SumI1OutMax=[]  SumI2OutMin=[]  SumI2OutMax=[]  SumI3OutMin=[]  SumI3OutMax=[]  SumDOutMin=[]  SumDOutMax=[]  SaturationOutMin=[]  SaturationOutMax=[]  IntegratorContinuousStateAttributes=''  IntegratorStateMustResolveToSignalObject=off  IntegratorRTWStateStorageClass=Auto  FilterContinuousStateAttributes=''  FilterStateMustResolveToSignalObject=off  FilterRTWStateStorageClass=Auto  DifferentiatorICPrevScaledInput=0  DifferentiatorOutMin=[]  DifferentiatorOutMax=[]
  PID Control Direction : simulink/Continuous/PID Controller  Controller=PID  TimeDomain=Discrete-time  SampleTime=Ts  IntegratorMethod=Forward Euler  FilterMethod=Forward Euler  Form=Parallel  UseFilter=on  ControllerParametersSource=internal  P=0.7  I=0.5  D=0  N=100  InitialConditionSource=internal  InitialConditionForIntegrator=0  InitialConditionForFilter=0  ExternalReset=none  LimitOutput=off  UpperSaturationLimit=inf  LowerSaturationLimit=-inf  LinearizeAsGain=on  AntiWindupMode=none  Kb=1  TrackingMode=off  Kt=1  PParamMin=[]  PParamMax=[]  IParamMin=[]  IParamMax=[]  DParamMin=[]  DParamMax=[]  NParamMin=[]  NParamMax=[]  KbParamMin=[]  KbParamMax=[]  KtParamMin=[]  KtParamMax=[]  POutMin=[]  POutMax=[]  IOutMin=[]  IOutMax=[]  DOutMin=[]  DOutMax=[]  NOutMin=[]  NOutMax=[]  KbOutMin=[]  KbOutMax=[]  KtOutMin=[]  KtOutMax=[]  IntegratorOutMin=[]  IntegratorOutMax=[]  FilterOutMin=[]  FilterOutMax=[]  SumOutMin=[]  SumOutMax=[]  SumI1OutMin=[]  SumI1OutMax=[]  SumI2OutMin=[]  SumI2OutMax=[]  SumI3OutMin=[]  SumI3OutMax=[]  SumDOutMin=[]  SumDOutMax=[]  SaturationOutMin=[]  SaturationOutMax=[]  IntegratorContinuousStateAttributes=''  IntegratorStateMustResolveToSignalObject=off  IntegratorRTWStateStorageClass=Auto  FilterContinuousStateAttributes=''  FilterStateMustResolveToSignalObject=off  FilterRTWStateStorageClass=Auto  DifferentiatorICPrevScaledInput=0  DifferentiatorOutMin=[]  DifferentiatorOutMax=[]
  PID Control Steering : simulink/Continuous/PID Controller  Controller=PID  TimeDomain=Discrete-time  SampleTime=Ts  IntegratorMethod=Forward Euler  FilterMethod=Forward Euler  Form=Parallel  UseFilter=on  ControllerParametersSource=internal  P=1  I=0.1  D=0  N=100  InitialConditionSource=internal  InitialConditionForIntegrator=0  InitialConditionForFilter=0  ExternalReset=none  LimitOutput=off  UpperSaturationLimit=inf  LowerSaturationLimit=-inf  LinearizeAsGain=on  AntiWindupMode=none  Kb=1  TrackingMode=off  Kt=1  PParamMin=[]  PParamMax=[]  IParamMin=[]  IParamMax=[]  DParamMin=[]  DParamMax=[]  NParamMin=[]  NParamMax=[]  KbParamMin=[]  KbParamMax=[]  KtParamMin=[]  KtParamMax=[]  POutMin=[]  POutMax=[]  IOutMin=[]  IOutMax=[]  DOutMin=[]  DOutMax=[]  NOutMin=[]  NOutMax=[]  KbOutMin=[]  KbOutMax=[]  KtOutMin=[]  KtOutMax=[]  IntegratorOutMin=[]  IntegratorOutMax=[]  FilterOutMin=[]  FilterOutMax=[]  SumOutMin=[]  SumOutMax=[]  SumI1OutMin=[]  SumI1OutMax=[]  SumI2OutMin=[]  SumI2OutMax=[]  SumI3OutMin=[]  SumI3OutMax=[]  SumDOutMin=[]  SumDOutMax=[]  SaturationOutMin=[]  SaturationOutMax=[]  IntegratorContinuousStateAttributes=''  IntegratorStateMustResolveToSignalObject=off  IntegratorRTWStateStorageClass=Auto  FilterContinuousStateAttributes=''  FilterStateMustResolveToSignalObject=off  FilterRTWStateStorageClass=Auto  DifferentiatorICPrevScaledInput=0  DifferentiatorOutMin=[]  DifferentiatorOutMax=[]
  Reference Position and Direction in Global CS with variable Look Ahead : Subsystem
  Sum4 : Sum  Inputs=+--
  Sum5 : Sum  Inputs=|+-
  Switch : Switch  Criteria=u2 > Threshold
  Switch1 : Switch  Criteria=u2 > Threshold
  Switch2 : Switch  Criteria=u2 > Threshold
  Reference Steering Angle : Outport
  wires:
  Lateral Error/1(Lateral Error) -> PID Control Lateral Position/1  "Lateral Error"
  Sum5/1 -> PID Control Steering/1  "Delta Error"
  Estimated Position/1 -> " "/2
  " "/1 -> Lateral Error/2(Position Error (X,Y))  "Position Error"
  Reference Position and Direction in Global CS with variable Look Ahead/2(Position (X,Y)) -> " "/1
  Reference Position and Direction in Global CS with variable Look Ahead/1(Psi Sigma) -> Lateral Error/1(Psi Sigma), Sum4/1
  Sum4/1 -> PID Control Direction/1  "Delta Reference = Psi Sigma - Nu"
  Measured Steering Angle/1 -> Gain/1
  Estimated Heading/1 -> Sum4/3
  Measured Velocity/1 -> Reference Position and Direction in Global CS with variable Look Ahead/1(Velocity)
  Gain/1 -> Sum5/2
  Switch/1 -> Switch1/3, Sum4/2
  PID Control Lateral Position/1 -> Switch/1
  Constant/1 -> Switch/2
  Switch1/1 -> Switch2/3, Sum5/1
  PID Control Direction/1 -> Switch1/1
  Constant1/1 -> Switch1/2
  PID Control Steering/1 -> Switch2/1  "Delta Reference"
  Switch2/1 -> Reference Steering Angle/1
  Constant2/1 -> Switch2/2

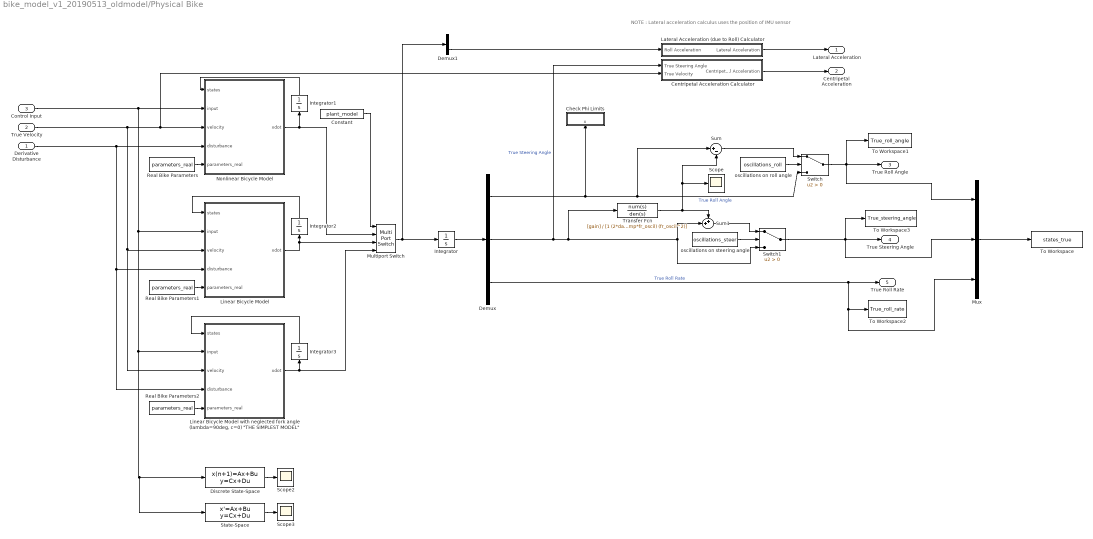
== system bike_model_v1_20190513_oldmodel/Physical Bike ==
  note: NOTE : Lateral acceleration calculus uses the position of IMU sensor
  Derivative Disturbance : Inport
  True Velocity : Inport  Port=2
  Control Input : Inport  Port=3
  Centripetal Acceleration Calculator : Subsystem
  Check Phi Limits : Subsystem  TreatAsAtomicUnit=on  SystemSampleTime=Ts
  Constant : Constant  Value=plant_model
  Demux : Demux  Outputs=3
  Demux1 : Demux  Outputs=3
  Discrete State-Space : DiscreteStateSpace  A=sys_dis.A  B=sys_dis.B  C=eye(3,3)  D=zeros(3,1)  SampleTime=Ts_IMU
  Integrator{,1..3} (4 alike) : Integrator  InitialCondition=initial_states
  Lateral Acceleration (due to Roll) Calculator : Subsystem
  Linear Bicycle Model : MATLAB Function  TreatAsAtomicUnit=on
  "Linear Bicycle Model with neglected fork angle (lambda=90deg, c=0) \"THE SIMPLEST MODEL\"" : MATLAB Function  TreatAsAtomicUnit=on
  Multiport Switch : MultiPortSwitch
  Mux : Mux  Inputs=3
  Nonlinear Bicycle Model : MATLAB Function  TreatAsAtomicUnit=on
  Real Bike Parameters : Constant  Value=parameters_real
  Real Bike Parameters1 : Constant  Value=parameters_real
  Real Bike Parameters2 : Constant  Value=parameters_real
  Scope : Scope
  Scope2 : Scope
  Scope3 : Scope
  State-Space : StateSpace  A=sys_con.A  B=sys_con.B  C=eye(3,3)  D=zeros(3,1)  X0=0
  Sum : Sum  Inputs=|+-
  Sum1 : Sum  Inputs=++|
  Switch : Switch  Criteria=u2 > Threshold
  Switch1 : Switch  Criteria=u2 > Threshold
  To Workspace : ToWorkspace  VariableName=states_true  SaveFormat=Timeseries  SampleTime=Ts
  To Workspace1 : ToWorkspace  VariableName=True_roll_angle  SaveFormat=Structure  SampleTime=Ts
  To Workspace2 : ToWorkspace  VariableName=True_roll_rate  SaveFormat=Structure  SampleTime=Ts
  To Workspace3 : ToWorkspace  VariableName=True_steering_angle  SaveFormat=Structure  SampleTime=-1
  Transfer Fcn : TransferFcn  Numerator=[gain]  Denominator=[1 (2*damp*fr_oscil) (fr_oscil^2)]
  "oscillations on roll angle " : Constant  Value=oscillations_roll
  oscillations on steering angle : Constant  Value=oscillations_steer
  Lateral Acceleration : Outport
  Centripetal Acceleration : Outport  Port=2
  True Roll Angle : Outport  Port=3
  True Steering Angle : Outport  Port=4
  True Roll Rate : Outport  Port=5
  wires:
  Derivative Disturbance/1 -> "Linear Bicycle Model with neglected fork angle (lambda=90deg, c=0) \"THE SIMPLEST MODEL\""/4(disturbance), Linear Bicycle Model/4(disturbance), Nonlinear Bicycle Model/4(disturbance)
  Centripetal Acceleration Calculator/1(Centripetal Acceleration) -> Centripetal Acceleration/1
  Lateral Acceleration (due to Roll) Calculator/1(Lateral Acceleration) -> Lateral Acceleration/1
  True Velocity/1 -> Centripetal Acceleration Calculator/2(True Velocity), Nonlinear Bicycle Model/3(velocity), "Linear Bicycle Model with neglected fork angle (lambda=90deg, c=0) \"THE SIMPLEST MODEL\""/3(velocity), Linear Bicycle Model/3(velocity)
  Demux/3 -> To Workspace2/1, Mux/3, True Roll Rate/1  "True Roll Rate"
  Real Bike Parameters/1 -> Nonlinear Bicycle Model/5(parameters_real)
  Nonlinear Bicycle Model/1(xdot) -> Integrator1/1, Multiport Switch/2
  Linear Bicycle Model/1(xdot) -> Integrator2/1, Multiport Switch/3
  Real Bike Parameters1/1 -> Linear Bicycle Model/5(parameters_real)
  Multiport Switch/1 -> Demux1/1, Integrator/1
  Constant/1 -> Multiport Switch/1
  "Linear Bicycle Model with neglected fork angle (lambda=90deg, c=0) \"THE SIMPLEST MODEL\""/1(xdot) -> Integrator3/1, Multiport Switch/4
  Real Bike Parameters2/1 -> "Linear Bicycle Model with neglected fork angle (lambda=90deg, c=0) \"THE SIMPLEST MODEL\""/5(parameters_real)
  Demux1/3 -> Lateral Acceleration (due to Roll) Calculator/1(Roll Acceleration)
  Integrator/1 -> Demux/1
  Integrator3/1 -> "Linear Bicycle Model with neglected fork angle (lambda=90deg, c=0) \"THE SIMPLEST MODEL\""/1(states)
  Integrator2/1 -> Linear Bicycle Model/1(states)
  Integrator1/1 -> Nonlinear Bicycle Model/1(states)
  Discrete State-Space/1 -> Scope2/1
  State-Space/1 -> Scope3/1
  Control Input/1 -> State-Space/1, Discrete State-Space/1, "Linear Bicycle Model with neglected fork angle (lambda=90deg, c=0) \"THE SIMPLEST MODEL\""/2(input), Linear Bicycle Model/2(input), Nonlinear Bicycle Model/2(input)
  Mux/1 -> To Workspace/1
  Sum/1 -> Switch/1
  Demux/2 -> Switch1/3, Sum1/2, Transfer Fcn/1, Centripetal Acceleration Calculator/1(True Steering Angle)  "True Steering Angle"
  Demux/1 -> Sum/1, Switch/3, Check Phi Limits/1(x)  "True Roll Angle"
  "oscillations on roll angle "/1 -> Switch/2
  Transfer Fcn/1 -> Sum1/1, Scope/1, Sum/2
  Switch/1 -> True Roll Angle/1, To Workspace1/1, Mux/1
  Sum1/1 -> Switch1/1
  Switch1/1 -> To Workspace3/1, True Steering Angle/1, Mux/2
  oscillations on steering angle/1 -> Switch1/2

== system bike_model_v1_20190513_oldmodel/Steering Encoder ==
  Steering Angle (State) : Inport
  Constant : Constant  Value=noise
  Noise on steering encoder : RandomNumber  Variance=noise_encoder  Seed=6  SampleTime=Ts
  Sum : Sum  Inputs=++|
  Switch : Switch  Criteria=u2 > Threshold
  Zero-Order Hold : ZeroOrderHold  SampleTime=Ts
  Steering Angle : Outport
  wires:
  Constant/1 -> Switch/2
  Sum/1 -> Switch/1
  Steering Angle (State)/1 -> Sum/2, Switch/3
  Switch/1 -> Zero-Order Hold/1
  Zero-Order Hold/1 -> Steering Angle/1
  Noise on steering encoder/1 -> Sum/1

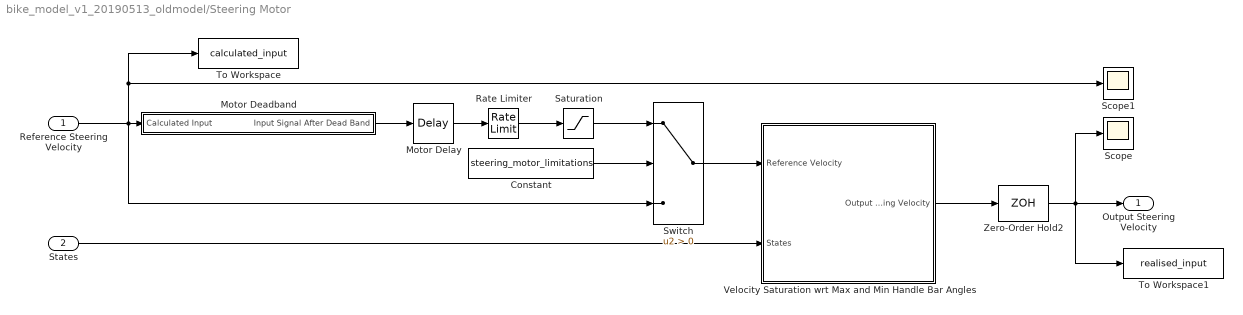
== system bike_model_v1_20190513_oldmodel/Steering Motor ==
  Reference Steering Velocity : Inport
  States : Inport  Port=2
  Constant : Constant  Value=steering_motor_limitations
  Motor Delay : TransportDelay  DelayTime=delay
  Motor Deadband : Subsystem
  Rate Limiter : RateLimiter  RisingSlewLimit=max_steering_motor_acc  FallingSlewLimit=min_steering_motor_acc  SampleTimeMode=inherited
  Saturation : Saturate  UpperLimit=max_steering_motor_speed  LowerLimit=min_steering_motor_speed
  Scope : Scope
  Scope1 : Scope
  Switch : Switch  Criteria=u2 > Threshold
  To Workspace : ToWorkspace  VariableName=calculated_input  SaveFormat=Timeseries  SampleTime=Ts
  To Workspace1 : ToWorkspace  VariableName=realised_input  SaveFormat=Timeseries  SampleTime=Ts
  Velocity Saturation wrt Max and Min Handle Bar Angles : Subsystem
  Zero-Order Hold2 : ZeroOrderHold  SampleTime=Ts
  Output Steering Velocity : Outport
  wires:
  States/1 -> Velocity Saturation wrt Max and Min Handle Bar Angles/2(States)
  Motor Delay/1 -> Rate Limiter/1
  Constant/1 -> Switch/2
  Switch/1 -> Velocity Saturation wrt Max and Min Handle Bar Angles/1(Reference Velocity)
  Rate Limiter/1 -> Saturation/1
  Saturation/1 -> Switch/1
  Velocity Saturation wrt Max and Min Handle Bar Angles/1(Output Steering Velocity) -> Zero-Order Hold2/1
  Motor Deadband/1(Input Signal After Dead Band) -> Motor Delay/1
  Zero-Order Hold2/1 -> To Workspace1/1, Scope/1, Output Steering Velocity/1
  Reference Steering Velocity/1 -> Scope1/1, To Workspace/1, Motor Deadband/1(Calculated Input), Switch/3

== system bike_model_v1_20190513_oldmodel/Velocity Reference ==
  note: If you will use this variable velocity
      | reference generator, you need to change
      | upper and lower limits of velocity specified
      | in initialization code!
  Add : Sum  Inputs=4
  Constant Velocity : Constant  Value=input_velocity
  Ramp : simulink/Sources/Ramp  slope=0.03  start=0  X0=0
  Reference Velocity Selector : ManualSwitch
  Sine Wave : Sin  Amplitude=0  SampleTime=0
  Step : Step  Time=20  Before=4  After=8  SampleTime=0
  Step1 : Step  Time=40  After=-1  SampleTime=0
  V_ref : Outport
  wires:
  Ramp/1 -> Add/4
  Constant Velocity/1 -> Reference Velocity Selector/1
  Step1/1 -> Add/3
  Step/1 -> Add/2
  Sine Wave/1 -> Add/1
  Add/1 -> Reference Velocity Selector/2
  Reference Velocity Selector/1 -> V_ref/1
